simulink model "main"  (R2019b)
settings: Solver=ode45  StartTime=0.0  StopTime=600  FixedStep=0.1  MaxStep=0.1  RelTol=1e-3
libraries: fuzblock x2
settings Model: Creator=hfekriaz  LastModifiedBy=hfekriaz
settings DataIOCC: ReturnWorkspaceOutputs=off
settings DebuggingCC: ArithmeticOperatorsInVariantConditions=warning
settings SFSimCC: SimUseLocalCustomCode=off  CustomCodeUndefinedFunction=UseInterfaceOnly
settings RTWCC: RTWUseLocalCustomCode=off

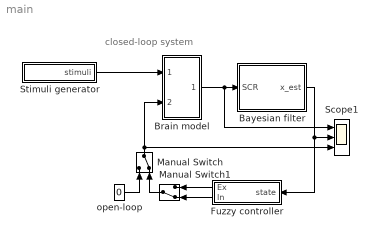
== system main ==
  note: closed-loop system
  Bayesian filter : Subsystem
  "Brain model " : Subsystem
  Fuzzy controller : Subsystem
  Manual Switch : ManualSwitch  CurrentSetting=0
  Manual Switch1 : ManualSwitch  CurrentSetting=0
  Scope1 : Scope  NumInputPorts=3
  "Stimuli generator " : Subsystem
  open-loop : Constant  Value=0
  wires:
  Bayesian filter/1(x_est) -> Fuzzy controller/1(state), Scope1/2
  Fuzzy controller/1("Ex ") -> Manual Switch1/1
  Fuzzy controller/2("In ") -> Manual Switch1/2
  "Stimuli generator "/1("stimuli ") -> "Brain model "/1(u_s)
  Manual Switch/1 -> "Brain model "/2(Control), Scope1/3
  "Brain model "/1("SCR ") -> Scope1/1, Bayesian filter/1(SCR)
  Manual Switch1/1 -> Manual Switch/2
  open-loop/1 -> Manual Switch/1

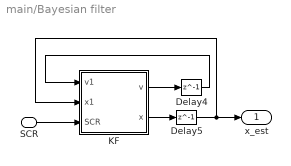
== system main/Bayesian filter ==
  SCR : Inport
  Delay4 : Delay  DelayLength=1  InitialCondition=0.000418027082743929
  Delay5 : Delay  DelayLength=1  InitialCondition=0.9
  KF : MATLAB Function  TreatAsAtomicUnit=on
  x_est : Outport  VectorParamsAs1DForOutWhenUnconnected=off
  wires:
  KF/2(x) -> Delay5/1
  KF/1(v) -> Delay4/1
  Delay4/1 -> KF/1(v1)
  Delay5/1 -> KF/2(x1), x_est/1
  SCR/1 -> KF/3(SCR)

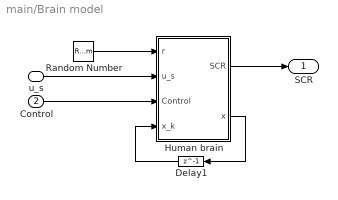
== system main/Brain model  ==
  u_s : Inport
  Control : Inport  Port=2
  Delay1 : Delay  DelayLength=1  InitialCondition=0.9
  Human brain : MATLAB Function  TreatAsAtomicUnit=on
  Random Number : RandomNumber  Variance=0.0001  Seed=52
  "SCR " : Outport  VectorParamsAs1DForOutWhenUnconnected=off
  wires:
  u_s/1 -> Human brain/2(u_s)
  Random Number/1 -> Human brain/1(r)
  Delay1/1 -> Human brain/4(x_k)
  Human brain/1(SCR) -> "SCR "/1
  Human brain/2(x) -> Delay1/1
  Control/1 -> Human brain/3(Control)

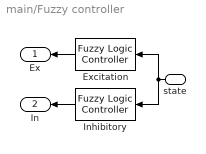
== system main/Fuzzy controller ==
  state : Inport
  Excitation : fuzblock/Fuzzy Logic  Controller  FIS='Ex.fis'  OutputSampleNumber=101  DataType=double  FuzzifiedInputs=off  RuleFiringStrengths=off  RuleOutputs=off  AggregatedOutputs=off  SimulateUsing=Interpreted execution  OutOfRangeInputValueMessage=warning  NoRuleFiredMessage=warning  EmptyOutputFuzzySetMessage=warning
  Inhibitory : fuzblock/Fuzzy Logic  Controller  FIS='In.fis'  OutputSampleNumber=101  DataType=double  FuzzifiedInputs=off  RuleFiringStrengths=off  RuleOutputs=off  AggregatedOutputs=off  SimulateUsing=Interpreted execution  OutOfRangeInputValueMessage=warning  NoRuleFiredMessage=warning  EmptyOutputFuzzySetMessage=warning
  "Ex " : Outport  VectorParamsAs1DForOutWhenUnconnected=off
  "In " : Outport  Port=2  VectorParamsAs1DForOutWhenUnconnected=off
  wires:
  state/1 -> Inhibitory/1, Excitation/1
  Excitation/1 -> "Ex "/1
  Inhibitory/1 -> "In "/1

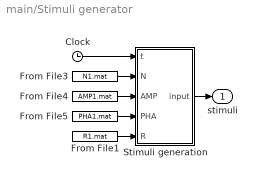
== system main/Stimuli generator  ==
  Clock : Clock
      settings: Decimation=10000
  From File1 : FromFile  FileName=R1.mat
  From File3 : FromFile  FileName=N1.mat
  From File4 : FromFile  FileName=AMP1.mat
  From File5 : FromFile  FileName=PHA1.mat
  Stimuli generation : MATLAB Function  TreatAsAtomicUnit=on
  "stimuli " : Outport  VectorParamsAs1DForOutWhenUnconnected=off
  wires:
  Clock/1 -> Stimuli generation/1(t)
  From File5/1 -> Stimuli generation/4(PHA)
  From File3/1 -> Stimuli generation/2(N)
  From File4/1 -> Stimuli generation/3(AMP)
  Stimuli generation/1(input) -> "stimuli "/1
  From File1/1 -> Stimuli generation/5(R)

== matlab function main/Bayesian filter/KF ==
  data: v1 input; v output; x1 input; x output; SCR input
function [v,x]= fcn(v1,x1,SCR)

n = SCR;
M = 1;
veps = zeros(1, M + 1);

%%% use the corresponding alpha value and veps_guess associated with each simulated profile
%%%% make sure to use the corresponding intial values for the blocks in the
%%%% Bayesian filter subsystem


%%%%% (1) x_0 = 0.9
alpha  = -1.9;
veps_guess =0.000418027082743929;

% %%%%% (2) x_0 = 0.4
% alpha  = -1.8;
% veps_guess =0.0008056270766531009;

% %%%%% (3) x_0 = 0.4
% alpha  = -1.95;
% veps_guess =0.0004190570765517610;

% %%%%% (4) x_0 = 0.4
% alpha  = -1.8;
% veps_guess =0.0003120210587517699;

% %%%%% (5) x_0 = 0.5
% alpha  = -1.95;
% veps_guess =0.0004212211587571931;

% %%%%% (6) x_0 = 0.7
% alpha  = -2.2;
% veps_guess =0.0001990211427517221;

veps(1) = veps_guess;
mu = -1.2;
tol = 10^(-14);

% chance_prob = sum(n) / length(n);
% N = length(n);
% mu = log(chance_prob / (1 - chance_prob));

v3 = v1 + veps(1);
vkj=v3;
xkj=x1;
nk=n;

it = zeros(45,1);
g= zeros(45,1);
gprime= zeros(45,1);
it(1) = xkj + vkj * (nk - exp(mu + xkj) / (1 + exp(mu + xkj)));
sol = 0;

for i = 1:40    
   g(i)     = xkj + vkj * (nk - exp(mu + it(i)) / (1 + exp(mu + it(i)))) - it(i);
   gprime(i)= (-1) * vkj * exp(mu + it(i)) / (1 + exp(mu + it(i)))^2 - 1;
   it(i+1)  = it(i) - g(i)/gprime(i);

   sol = it(i+1);
   
   if abs(sol - it(i))>tol 
      continue 
   end
end 
x = sol;
v = ((1 / (v3)) + (exp(mu + x)) / ((1 + exp(mu + x))*(1 / (1 + exp(mu + x)))))^(-1);
% v = 1 / ((1 / (v3)) + (exp(mu + x) / (1 + exp(mu + x))) ...
%     * (1 / (1 + exp(mu + x)))); 

q = 1/(1+exp(-1*(alpha +x)));
s=0;
if q>rand(1)
    s = 1;
end

end

== matlab function main/Brain model /Human brain ==
  settings: updateMethod=DISCRETE
  data: r input; u_s input; Control input; SCR output; x output; x_k input
function [SCR,x]  = fcn(r,u_s,Control,x_k)

x = x_k + u_s + Control + r ;


%%% Initial value and alpha parametr asscoitaed with each six simulated
%%% profiles (use the corresponding alpha value for this block) (use the initila value in the brain model block)

%%%%% (1) x_0 = 0.9
alpha  = -1.9;

% %%%%% (2) x_0 = 0.4
% alpha  = -1.8;

% %%%%% (3) x_0 = 0.4
% alpha  = -1.95;

% %%%%% (4) x_0 = 0.4
% alpha  = -1.8;

% %%%%% (5) x_0 = 0.5
% alpha  = -1.95;

% %%%%% (6) x_0 = 0.7
% alpha  = -2.2;



q = 1/(1+exp(-1*(alpha +x))); %%%% Bernouli Distribution 
SCR=0;
if rand(1)<q
    SCR = 1;
end

end

== matlab function main/Stimuli generator /Stimuli generation ==
  data: t input; N input; AMP input; PHA input; input output; R input
function input = fcn(t,N,AMP,PHA,R)
%%%% for other subject, make sure to change the numbers in the
%%%% corresponding blocks (i.e., N,AMP,PHA,R)
a =R(1,1);
b =R(2,1);
c =R(3,1);
d =R(4,1);
T1 = 300;
if t < T1 %%% high arousal stimuli 
    Y1 = 0;
    for i=1:length(N)
        Y1 = AMP(i)*cos(N(i)*t + PHA(i)) + Y1 ;
    end
    input = Y1;
else      %%%% low arousal stimuli
    input  =  a*exp(b*(t-T1)) + c*exp(d*(t-T1));
end
end
